simulink model "HDL_Code"  (R2023a)
settings: Solver=FixedStepAuto  StartTime=0.0  StopTime=5  RelTol=1e-3
settings Model: Creator=Tien  LastModifiedBy=Tien
settings DebuggingCC: ParameterPrecisionLossMsg=none

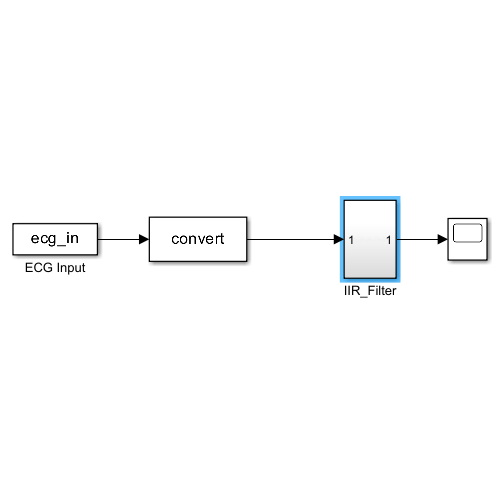
[thumbnail: Simulink's stored preview of the top-level diagram]
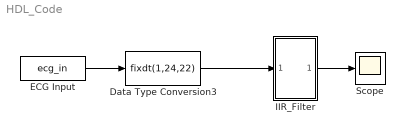
== system HDL_Code ==
  Data Type Conversion3 : DataTypeConversion  OutDataTypeStr=fixdt(1,24,22)  RndMeth=Round
  ECG Input : FromWorkspace  VariableName=ecg_in  SampleTime=0.002
  IIR_Filter : Subsystem
  Scope : Scope
  wires:
  ECG Input/1 -> Data Type Conversion3/1
  Data Type Conversion3/1 -> IIR_Filter/1(In1)
  IIR_Filter/1(Out1) -> Scope/1

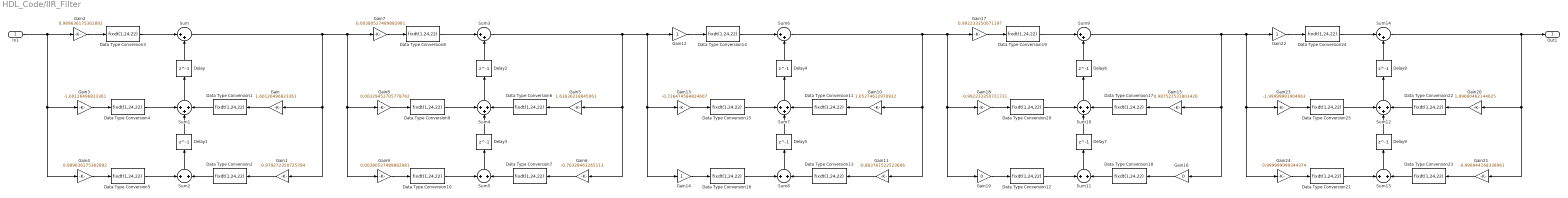
== system HDL_Code/IIR_Filter ==
  In1 : Inport  OutDataTypeStr=fixdt(1,24,22)
  Data Type Conversion{1..25} (25 alike) : DataTypeConversion  OutDataTypeStr=fixdt(1,24,22)  RndMeth=Round
  Delay{,1..9} (10 alike) : Delay  DelayLength=1  InitialCondition=0
  Gain : Gain  Gain=1.60126496823361  RndMeth=Round  SaturateOnIntegerOverflow=on
  Gain1 : Gain  Gain=-0.979272350725784
  Gain10 : Gain  Gain=1.65274612970922  RndMeth=Round  SaturateOnIntegerOverflow=on
  Gain11 : Gain  Gain=-0.883761522523606
  Gain12 : Gain  RndMeth=Nearest
  Gain13 : Gain  Gain=-0.736474584824607  RndMeth=Round
  Gain14 : Gain
  Gain15 : Gain  Gain=0.987522531803426  RndMeth=Round  SaturateOnIntegerOverflow=on
  Gain16 : Gain  Gain=0
  Gain17 : Gain  Gain=0.992233350071197  RndMeth=Nearest
  Gain18 : Gain  Gain=-0.992233350721731  RndMeth=Round
  Gain19 : Gain  Gain=0
  Gain2 : Gain  Gain=0.989636175362892  RndMeth=Nearest
  Gain20 : Gain  Gain=1.99690462144625  RndMeth=Round  SaturateOnIntegerOverflow=on
  Gain21 : Gain  Gain=-0.996944168338961
  Gain22 : Gain  RndMeth=Nearest
  Gain23 : Gain  Gain=-1.99999881904963  RndMeth=Round
  Gain24 : Gain  Gain=0.999999999344374
  Gain3 : Gain  Gain=-1.60126496823361  RndMeth=Round
  Gain4 : Gain  Gain=0.989636175362892
  Gain5 : Gain  Gain=1.63636218845061  RndMeth=Round  SaturateOnIntegerOverflow=on
  Gain6 : Gain  Gain=-0.70328463265113
  Gain7 : Gain  Gain=0.00380527489882981  RndMeth=Nearest
  Gain8 : Gain  Gain=0.00329452705778762  RndMeth=Round
  Gain9 : Gain  Gain=0.00380527489882981
  Sum{,3,6,9,14} (5 alike) : Sum  Inputs=|++  OutDataTypeStr=fixdt(1,40,30)  RndMeth=Round  SaturateOnIntegerOverflow=on
  Sum{1,4,7,10,12} (5 alike) : Sum  Inputs=+++  OutDataTypeStr=fixdt(1,40,30)  RndMeth=Round  SaturateOnIntegerOverflow=on
  Sum{2,5,8,11,13} (5 alike) : Sum  Inputs=+|+  OutDataTypeStr=fixdt(1,40,30)  RndMeth=Round  SaturateOnIntegerOverflow=on
  Out1 : Outport  OutDataTypeStr=fixdt(1,40,30)
  wires:
  Gain4/1 -> Data Type Conversion5/1
  In1/1 -> Gain4/1, Gain3/1, Gain2/1
  Delay1/1 -> Sum1/2
  Data Type Conversion5/1 -> Sum2/1
  Delay/1 -> Sum/2
  Data Type Conversion1/1 -> Sum1/3
  Sum1/1 -> Delay/1
  Gain/1 -> Data Type Conversion1/1
  Data Type Conversion3/1 -> Sum/1
  Gain1/1 -> Data Type Conversion2/1
  Data Type Conversion2/1 -> Sum2/2
  Sum2/1 -> Delay1/1
  Gain2/1 -> Data Type Conversion3/1
  Gain3/1 -> Data Type Conversion4/1
  Data Type Conversion4/1 -> Sum1/1
  Gain6/1 -> Data Type Conversion7/1
  Data Type Conversion9/1 -> Sum4/1
  Gain8/1 -> Data Type Conversion9/1
  Gain9/1 -> Data Type Conversion10/1
  Sum5/1 -> Delay3/1
  Gain7/1 -> Data Type Conversion8/1
  Delay3/1 -> Sum4/2
  Data Type Conversion7/1 -> Sum5/2
  Data Type Conversion8/1 -> Sum3/1
  Sum4/1 -> Delay2/1
  Data Type Conversion10/1 -> Sum5/1
  Gain5/1 -> Data Type Conversion6/1
  Data Type Conversion6/1 -> Sum4/3
  Sum/1 -> Gain9/1, Gain8/1, Gain7/1, Gain1/1, Gain/1
  Delay2/1 -> Sum3/2
  Sum10/1 -> Delay6/1
  Sum11/1 -> Delay7/1
  Data Type Conversion19/1 -> Sum9/1
  Data Type Conversion17/1 -> Sum10/3
  Gain15/1 -> Data Type Conversion17/1
  Delay6/1 -> Sum9/2
  Data Type Conversion20/1 -> Sum10/1
  Gain11/1 -> Data Type Conversion13/1
  Data Type Conversion15/1 -> Sum7/1
  Gain13/1 -> Data Type Conversion15/1
  Gain16/1 -> Data Type Conversion18/1
  Gain14/1 -> Data Type Conversion16/1
  Sum8/1 -> Delay5/1
  Gain12/1 -> Data Type Conversion14/1
  Gain19/1 -> Data Type Conversion12/1
  Delay5/1 -> Sum7/2
  Sum6/1 -> Gain19/1, Gain18/1, Gain17/1, Gain11/1, Gain10/1
  Data Type Conversion13/1 -> Sum8/2
  Data Type Conversion14/1 -> Sum6/1
  Data Type Conversion12/1 -> Sum11/1
  Sum7/1 -> Delay4/1
  Data Type Conversion16/1 -> Sum8/1
  Gain10/1 -> Data Type Conversion11/1
  Data Type Conversion11/1 -> Sum7/3
  Sum3/1 -> Gain14/1, Gain13/1, Gain12/1, Gain6/1, Gain5/1
  Gain18/1 -> Data Type Conversion20/1
  Delay4/1 -> Sum6/2
  Data Type Conversion18/1 -> Sum11/2
  Gain17/1 -> Data Type Conversion19/1
  Delay7/1 -> Sum10/2
  Gain21/1 -> Data Type Conversion23/1
  Delay8/1 -> Sum14/2
  Sum12/1 -> Delay8/1
  Data Type Conversion24/1 -> Sum14/1
  Data Type Conversion22/1 -> Sum12/3
  Sum13/1 -> Delay9/1
  Data Type Conversion25/1 -> Sum12/1
  Gain20/1 -> Data Type Conversion22/1
  Gain24/1 -> Data Type Conversion21/1
  Gain23/1 -> Data Type Conversion25/1
  Data Type Conversion23/1 -> Sum13/2
  Sum14/1 -> Out1/1, Gain21/1, Gain20/1
  Data Type Conversion21/1 -> Sum13/1
  Gain22/1 -> Data Type Conversion24/1
  Delay9/1 -> Sum12/2
  Sum9/1 -> Gain24/1, Gain23/1, Gain22/1, Gain16/1, Gain15/1
